simulink model "EX1"  (R2021b)
settings: Solver=VariableStepAuto  StartTime=0.0  StopTime=10  RelTol=1e-3
libraries: simulink x5
settings Model: Creator=Venik  LastModifiedBy=Venik

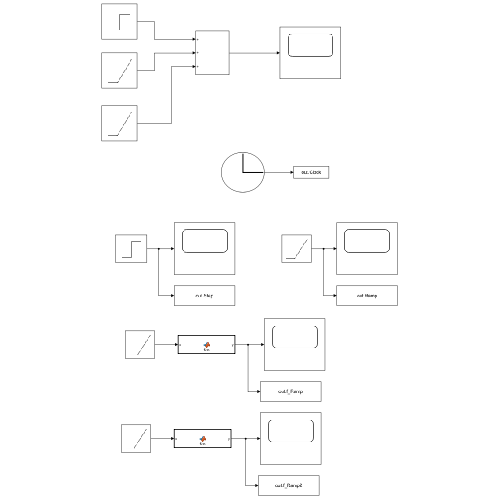
[thumbnail: Simulink's stored preview of the top-level diagram]
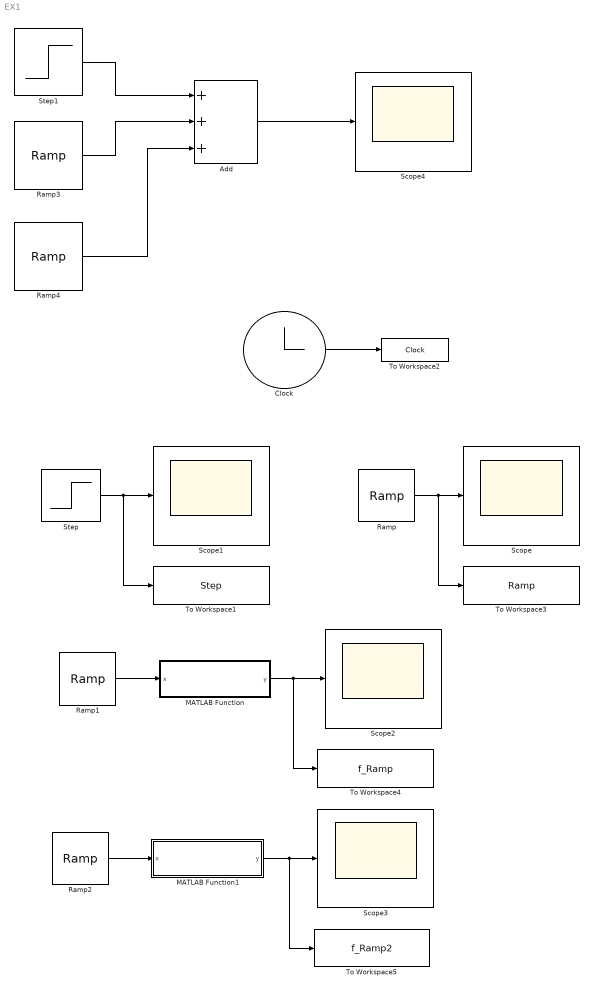
== system EX1 ==
  Add : Sum  Inputs=+++
  Clock : Clock
  MATLAB Function : MATLAB Function  TreatAsAtomicUnit=on
  MATLAB Function1 : MATLAB Function  TreatAsAtomicUnit=on
  Ramp : simulink/Sources/Ramp  slope=0.5  start=5  InitialOutput=1
  Ramp1 : simulink/Sources/Ramp  slope=1  start=0  InitialOutput=-3
  Ramp2 : simulink/Sources/Ramp  slope=1  start=0  InitialOutput=-3
  Ramp3 : simulink/Sources/Ramp  slope=-1  start=2  InitialOutput=2
  Ramp4 : simulink/Sources/Ramp  slope=1  start=4  InitialOutput=0
  Scope{,1..4} (5 alike) : Scope
  Step : Step  Time=5  Before=1  After=2  SampleTime=0
  Step1 : Step  Before=-1  After=0  SampleTime=0
  To Workspace1 : ToWorkspace  VariableName=Step  SampleTime=-1
  To Workspace2 : ToWorkspace  VariableName=Clock  SampleTime=-1
  To Workspace3 : ToWorkspace  VariableName=Ramp  SampleTime=-1
  To Workspace4 : ToWorkspace  VariableName=f_Ramp  SampleTime=-1
  To Workspace5 : ToWorkspace  VariableName=f_Ramp2  SampleTime=-1
  wires:
  Ramp/1 -> To Workspace3/1, Scope/1
  Step/1 -> To Workspace1/1, Scope1/1
  Clock/1 -> To Workspace2/1
  Ramp1/1 -> MATLAB Function/1(x)
  Ramp2/1 -> MATLAB Function1/1(x)
  MATLAB Function1/1(y) -> To Workspace5/1, Scope3/1
  MATLAB Function/1(y) -> To Workspace4/1, Scope2/1
  Ramp3/1 -> Add/2
  Step1/1 -> Add/1
  Add/1 -> Scope4/1
  Ramp4/1 -> Add/3

== matlab function EX1/MATLAB Function ==
  data: x input; y output
function y = fcn(x)

y = 2.*x.*x + 5.*x +1;

== matlab function EX1/MATLAB Function1 ==
  data: x input; y output
function y = fcn(x)

y = 2.*exp(2.*x) + exp(x) + 3;
